simulink model "globalPlanServer"  (R2024a)
settings: Solver=FixedStepAuto  StartTime=0.0  StopTime=inf  RelTol=1e-3
model workspace (MAT data in the model file):
  SL_ROS_VariableLengthArrays_MaxSizes.CommonInfo.ArrayTruncateAction = 'EmitWarning'
  SL_ROS_VariableLengthArrays_MaxSizes.MsgTypeMap = containers.Map
  SL_ROS_VariableLengthArrays_MaxSizes.MsgTypeMap.serialization.keys = {'std_msgs/Float64MultiArray'}
  SL_ROS_VariableLengthArrays_MaxSizes.MsgTypeMap.serialization.values{1}.PropertyName = 'data'
  SL_ROS_VariableLengthArrays_MaxSizes.MsgTypeMap.serialization.values{1}.DataType = 'double'
  SL_ROS_VariableLengthArrays_MaxSizes.MsgTypeMap.serialization.values{1}.MaxLength = 1500000
  SL_ROS_VariableLengthArrays_MaxSizes.MsgTypeMap.serialization.uniformity = 0
  SL_ROS_VariableLengthArrays_MaxSizes.MsgTypeMap.serialization.keyType = 'char'
  SL_ROS_VariableLengthArrays_MaxSizes.MsgTypeMap.serialization.valueType = 'any'
libraries: ros2lib x2, roshelperlib x2, simulink x1
settings Model: Creator=cstabile  LastModifiedBy=cstabile
settings OptimizationCC: EnhancedBackFolding=on  PassReuseOutputArgsAs=Individual arguments  ZeroExternalMemoryAtStartup=off  ZeroInternalMemoryAtStartup=off  MaxStackSize=64  OptimizeBlockOrder=speed  DifferentSizesBufferReuse=on  OptimizationCustomize=off  EfficientTunableParamExpr=on
settings DebuggingCC: ParameterTunabilityLossMsg=error
settings SFSimCC: MATLABDynamicMemAlloc=off
settings RTWCC: Description=Embedded Coder  SystemTargetFile=ert.tlc  HardwareBoard=Robot Operating System 2 (ROS 2)  TLCOptions="-aInlineSetEventsForThisBaseRateFcn=TLC_FALSE -aSuppressMultiTaskScheduler=TLC_FALSE  -aRateBasedStepFcn=0"  TemplateMakefile=ert_default_tmf  Toolchain=Colcon Tools  TargetLang=C++
settings CodeAppCC: ForceParamTrailComments=on  IgnoreCustomStorageClasses=off  OperatorAnnotations=on  SimulinkDataObjDesc=on  SFDataObjDesc=on  InsertBlockDesc=on
settings ERTTargetCC: CodeInterfacePackaging=C++ class  RootIOFormat=Structure reference

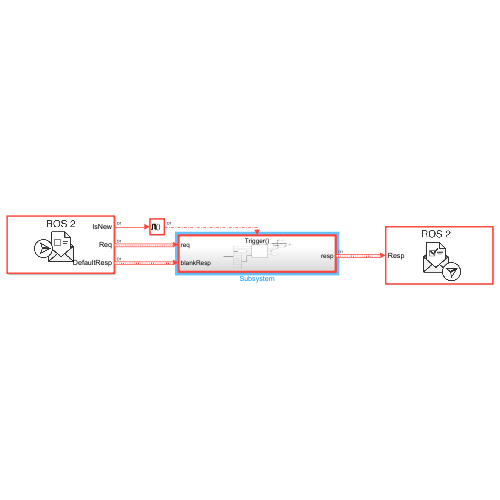
[thumbnail: Simulink's stored preview of the top-level diagram]
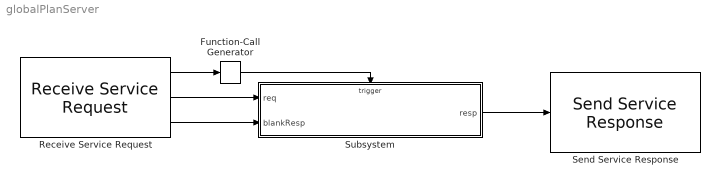
== system globalPlanServer ==
  Function-Call Generator : simulink/Ports & Subsystems/Function-Call Generator  sample_time=1  numberOfIterations=1  DisallowWideOutput=off  ShowEnablePort=on
  Receive Service Request : ros2lib/Receive Service Request  service=/planGlobal  serviceType=offroad_msg/PlanGlobal  SampleTime=-1  ShowDefaultRespOutput=on  BlockId=ServRec_globalPlanServer_1  QOSHistory=Keep last  QOSDepth=1  QOSReliability=Reliable  QOSDurability=Volatile  QOSDeadline=Inf  QOSLifespan=Inf  QOSLiveliness=Automatic  QOSLeaseDuration=Inf  QOSAvoidROSNamespaceConventions=off
      settings: LibrarySourceBlock=ros2lib/Receive Request
  Send Service Response : ros2lib/Send Service Response  service=/planGlobal  serviceType=offroad_msg/PlanGlobal  BlockId=ServRec_globalPlanServer_1
      settings: LibrarySourceBlock=ros2lib/Send Response
  Subsystem : Subsystem
  wires:
  Receive Service Request/1 -> Function-Call Generator/1
  Function-Call Generator/1 -> Subsystem/Trigger
  Receive Service Request/2 -> Subsystem/1(req)
  Receive Service Request/3 -> Subsystem/2(blankResp)
  Subsystem/1(resp) -> Send Service Response/1

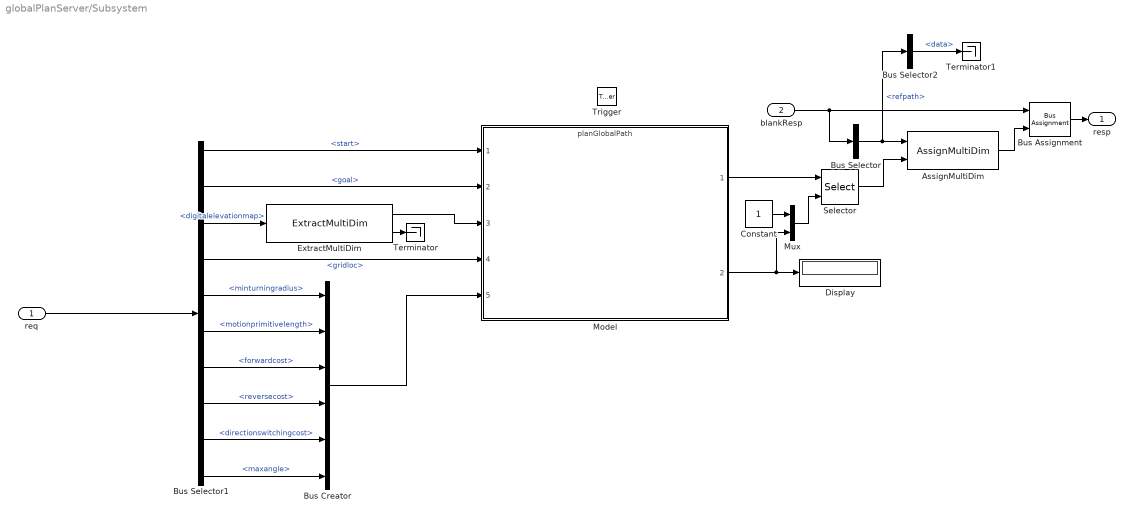
== system globalPlanServer/Subsystem ==
  req : Inport
  blankResp : Inport  Port=2
  Trigger : TriggerPort  TriggerType=function-call  VariantControl=(inherit)  PortDimensions=1
  AssignMultiDim : roshelperlib/AssignMultiDim  SystemSampleTime=-1  VariantActivationTime=update diagram  AllowFlexibleInterface=on  Latency=0  AutoFrameSizeCalculation=off
  Bus Assignment : BusAssignment  AssignedSignals=refpath
  Bus Creator : BusCreator  Inputs=6  OutDataTypeStr=Bus: fsp_tunable_bus
  Bus Selector : BusSelector  OutputSignals=refpath
  Bus Selector1 : BusSelector  OutputSignals=start,goal,digitalelevationmap,gridloc,tuneableterrainawareparams.minturningradius,tuneableterrainawareparams.motionprimitivelength,tuneableterrainawareparams.forwardcost,tuneableterrainawareparams.reversecost,tuneableterrainawareparams.directionswitchingcost,tuneableterrainawareparams.maxangle
  Bus Selector2 : BusSelector  OutputSignals=data
  Constant : Constant
  Display : Display
  ExtractMultiDim : roshelperlib/ExtractMultiDim  userDataType=single  dims=[1201 1201]  isVarsize=off  varsizeDims=[]  returnFixedTF=off
  Model : ModelReference  ModelNameDialog=planGlobalPath.slx  SimulationMode=Normal  ModelReferenceVersion=1.0
  Mux : Mux  Inputs=2
  Selector : Selector  NumberOfDimensions=2  InputPortWidth=3  IndexOptions=Starting and ending indices (port),Select all  Indices=[1 3],1  OutputSizes=1,1
  Terminator : Terminator
  Terminator1 : Terminator
  resp : Outport
  wires:
  Model/2 -> Mux/2, Display/1
  Model/1 -> Selector/1
  Constant/1 -> Mux/1
  Mux/1 -> Selector/2
  Bus Assignment/1 -> resp/1
  req/1 -> Bus Selector1/1
  Bus Selector1/1 -> Model/1  "<start>"
  Bus Selector1/2 -> Model/2  "<goal>"
  Bus Selector1/3 -> ExtractMultiDim/1  "<digitalelevationmap>"
  Bus Selector1/4 -> Model/4  "<gridloc>"
  blankResp/1 -> Bus Selector/1, Bus Assignment/1
  Selector/1 -> AssignMultiDim/2
  AssignMultiDim/1 -> Bus Assignment/2
  ExtractMultiDim/2 -> Terminator/1
  ExtractMultiDim/1 -> Model/3
  Bus Selector1/5 -> Bus Creator/1  "<minturningradius>"
  Bus Selector1/6 -> Bus Creator/2  "<motionprimitivelength>"
  Bus Selector1/7 -> Bus Creator/3  "<forwardcost>"
  Bus Selector1/8 -> Bus Creator/4  "<reversecost>"
  Bus Selector1/9 -> Bus Creator/5  "<directionswitchingcost>"
  Bus Selector1/10 -> Bus Creator/6  "<maxangle>"
  Bus Creator/1 -> Model/5
  Bus Selector/1 -> Bus Selector2/1, AssignMultiDim/1  "<refpath>"
  Bus Selector2/1 -> Terminator1/1  "<data>"
